simulink model "model33"  (R2019b)
settings: Solver=VariableStepAuto  StartTime=0.0  StopTime=10  RelTol=1e-3
settings Model: Creator=Já  LastModifiedBy=Já

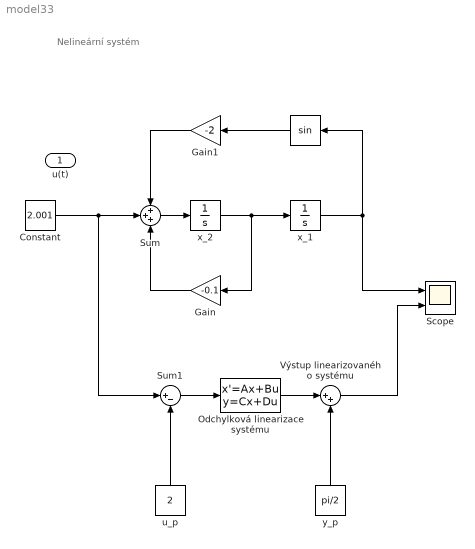
== system model33 ==
  note: Nelineární systém
  u(t) : Inport
  " " : Trigonometry
  Constant : Constant  Value=2.001
  Gain : Gain  Gain=-0.1
  Gain1 : Gain  Gain=-2
  Odchylková linearizace systému : StateSpace  A=[0 1; 0 -0.1]  B=[0;1]  C=[1 0]  D=0  InitialCondition=[0 ;0]
  Scope : Scope  NumInputPorts=2
  Sum : Sum  Inputs=+++
  Sum1 : Sum  Inputs=|+-
  Výstup linearizovaného systému : Sum  Inputs=|++
  u_p : Constant  Value=2
  x_1 : Integrator  InitialCondition=pi/2
  x_2 : Integrator
  y_p : Constant  Value=pi/2
  wires:
  x_2/1 -> x_1/1, Gain/1
  " "/1 -> Gain1/1
  Gain1/1 -> Sum/1
  Gain/1 -> Sum/3
  Sum/1 -> x_2/1
  x_1/1 -> Scope/1, " "/1
  Constant/1 -> Sum1/1, Sum/2
  Sum1/1 -> Odchylková linearizace systému/1
  Odchylková linearizace systému/1 -> Výstup linearizovaného systému/1
  Výstup linearizovaného systému/1 -> Scope/2
  y_p/1 -> Výstup linearizovaného systému/2
  u_p/1 -> Sum1/2
